simulink model "exsim2model"  (Simulink 8.6)
settings: Solver=ode45  StartTime=0.0  StopTime=tf  FixedStep=T  RelTol=1e-3
values from neighbouring files (symbols this model uses):
  a = 7/(4*T)    [controller.m]    (also in exsim2script.m = 2; exsim5script.m = 2)
  a1 = 7/(4*T)    (= 1.25)    [exsim2script.m]
  b = 2/(5*T)    [controller.m]    (also in exsim2script.m = 0.5; exsim5script.m = 0.5)
  b1 = 2/(5*T)    (= 0.285714285714)    [exsim2script.m]
  J = 1    [exsim2script.m]    (also in exsim5script.m)
  kc = 5/(4*alpha)    [controller.m]    (also in exsim2script.m = 2; exsim5script.m = 2)
  kc1 = 5/(4*alpha)    (= 1.27551020408)    [exsim2script.m]
  kp = 1    [exsim2script.m]    (also in exsim5script.m)
  r1 = 0.75    [controller2.m]    (also in ctrld.m; exsim2script.m; exsim5script.m)
  s0 = 1.25/alpha    [controller2.m]    (also in ctrld.m; exsim2script.m = 1.27551020408; exsim5script.m = 1.27551020408)
  s1 = -0.75/alpha    [controller2.m]    (also in ctrld.m; exsim2script.m = -0.765306122449; exsim5script.m = -0.765306122449)
  T = 1.4/w0    (= 1.4)    [exsim2script.m]    (also in exsim5script.m)
  t0 = 1/(2*alpha)    [controller2.m]    (also in ctrld.m; exsim2script.m = 0.510204081633; exsim5script.m = 0.510204081633)
settings Model: Creator=hcf2k  LastModifiedBy=hcf2k
settings DataIOCC: SaveFormat=StructureWithTime
settings OptimizationCC: ExpressionDepthLimit=128
settings DebuggingCC: UnderspecifiedInitializationDetection=Simplified  MergeDetectMultiDrivingBlocksExec=error  SolverPrmCheckMsg=none  FcnCallInpInsideContextMsg=EnableAllAsWarning  StateNameClashWarn=none
settings HardwareCC: ProdIntDivRoundTo=Zero  ProdEndianess=LittleEndian  ProdHWDeviceType=Specified
settings GRTTargetCC: GeneratePreprocessorConditionals=Use local settings
settings ConfigComp: CovModelRefEnable=off

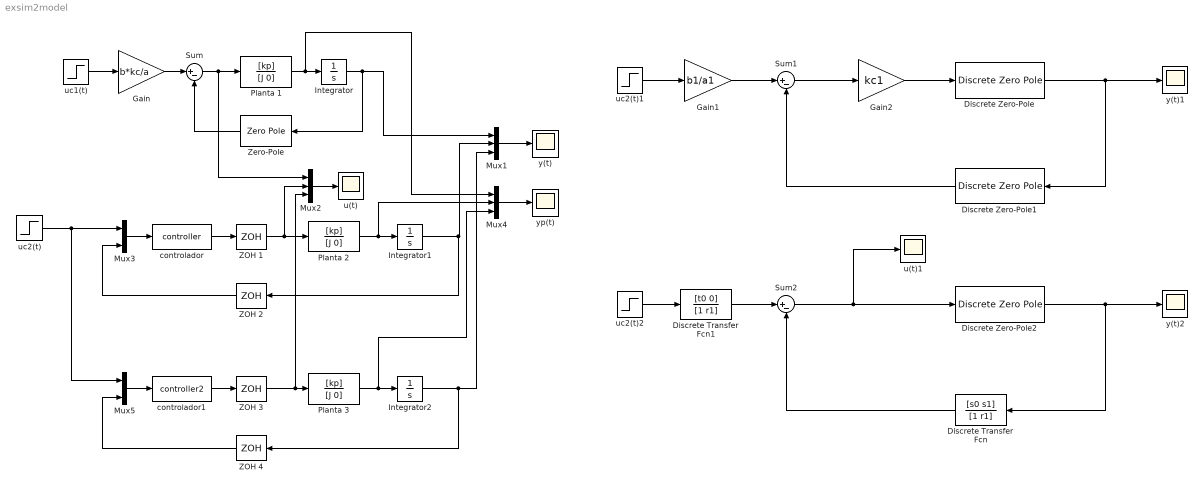
== system exsim2model ==
  Discrete Transfer Fcn : DiscreteTransferFcn  Numerator=[s0 s1]  Denominator=[1 r1]
  Discrete Transfer Fcn1 : DiscreteTransferFcn  Numerator=[t0 0]  Denominator=[1 r1]
  Discrete Zero-Pole : DiscreteZeroPole  Zeros=[-1]  Poles=[1 1]  Gain=kp*T^2/(2*J)  SampleTime=T
  Discrete Zero-Pole1 : DiscreteZeroPole  Zeros=[(1-b1*T)]  Poles=[(1-a1*T)]  Gain=1  SampleTime=T
  Discrete Zero-Pole2 : DiscreteZeroPole  Zeros=[-1]  Poles=[1 1]  Gain=kp*T^2/(2*J)  SampleTime=T
  Gain : Gain  Gain=b*kc/a
  Gain1 : Gain  Gain=b1/a1
  Gain2 : Gain  Gain=kc1
  Integrator : Integrator
  Integrator1 : Integrator
  Integrator2 : Integrator
  Mux1 : Mux  Inputs=3
  Mux2 : Mux  Inputs=3
  Mux3 : Mux  Inputs=2
  Mux4 : Mux  Inputs=3
  Mux5 : Mux  Inputs=2
  Planta 1 : TransferFcn  Numerator=[kp]  Denominator=[J 0]
  Planta 2 : TransferFcn  Numerator=[kp]  Denominator=[J 0]
  Planta 3 : TransferFcn  Numerator=[kp]  Denominator=[J 0]
  Sum : Sum  Inputs=|+-
  Sum1 : Sum  Inputs=|+-
  Sum2 : Sum  Inputs=|+-
  ZOH {1..4} (4 alike) : ZeroOrderHold  SampleTime=T
  Zero-Pole : ZeroPole  Zeros=[-b]  Poles=[-a]  Gain=[kc]
  controlador : MATLABFcn  MATLABFcn=controller  OutputDimensions=1
  controlador1 : MATLABFcn  MATLABFcn=controller2  OutputDimensions=1
  u(t) : Scope
  u(t)1 : Scope
  uc1(t) : Step  Time=0  SampleTime=0
  uc2(t) : Step  Time=0  SampleTime=T
  uc2(t)1 : Step  Time=0  SampleTime=T
  uc2(t)2 : Step  Time=0  SampleTime=T
  y(t) : Scope
  y(t)1 : Scope
  y(t)2 : Scope
  yp(t) : Scope
  wires:
  Mux1/1 -> y(t)/1
  Mux2/1 -> u(t)/1
  controlador/1 -> ZOH 1/1
  ZOH 1/1 -> Planta 2/1, Mux2/2
  Sum/1 -> Planta 1/1, Mux2/1
  Mux3/1 -> controlador/1
  Gain/1 -> Sum/1
  Zero-Pole/1 -> Sum/2
  ZOH 2/1 -> Mux3/2
  uc1(t)/1 -> Gain/1
  uc2(t)1/1 -> Gain1/1
  Gain1/1 -> Sum1/1
  Sum1/1 -> Gain2/1
  Gain2/1 -> Discrete Zero-Pole/1
  Discrete Zero-Pole1/1 -> Sum1/2
  Discrete Zero-Pole/1 -> Discrete Zero-Pole1/1, y(t)1/1
  Integrator/1 -> Zero-Pole/1, Mux1/1
  Planta 2/1 -> Mux4/2, Integrator1/1
  Integrator1/1 -> ZOH 2/1, Mux1/2
  Mux4/1 -> yp(t)/1
  Planta 1/1 -> Mux4/1, Integrator/1
  controlador1/1 -> ZOH 3/1
  ZOH 3/1 -> Mux2/3, Planta 3/1
  Mux5/1 -> controlador1/1
  ZOH 4/1 -> Mux5/2
  uc2(t)/1 -> Mux3/1, Mux5/1
  Planta 3/1 -> Mux4/3, Integrator2/1
  Integrator2/1 -> Mux1/3, ZOH 4/1
  uc2(t)2/1 -> Discrete Transfer Fcn1/1
  Discrete Transfer Fcn1/1 -> Sum2/1
  Sum2/1 -> u(t)1/1, Discrete Zero-Pole2/1
  Discrete Transfer Fcn/1 -> Sum2/2
  Discrete Zero-Pole2/1 -> Discrete Transfer Fcn/1, y(t)2/1
